simulink model "DC_Motor_Speed_Feedback_Controller"  (R2019b)
settings: Solver=FixedStepAuto  StartTime=0.0  StopTime=500  FixedStep=0.02  RelTol=1e-3  EnableMultiTasking=on
libraries: simulink x1, RoboholicLib x1, arduinolib x1
settings Model: SimulationMode=external  ExtModeTrigDuration=2  Creator=nbibin001  LastModifiedBy=ganna
settings DataIOCC: ReturnWorkspaceOutputs=off
settings OptimizationCC: PassReuseOutputArgsAs=Individual arguments  MaxStackSize=64  EfficientTunableParamExpr=on
settings DebuggingCC: ParameterTunabilityLossMsg=error  ArithmeticOperatorsInVariantConditions=warning
settings HardwareCC: ProdBitPerInt=16  ProdBitPerPointer=16  ProdBitPerSizeT=16  ProdBitPerPtrDiffT=16  ProdLargestAtomicFloat=None  ProdWordSize=8  ProdHWDeviceType=Atmel->AVR
settings SFSimCC: SimUseLocalCustomCode=off  MATLABDynamicMemAlloc=off  CustomCodeUndefinedFunction=UseInterfaceOnly
settings RTWCC: SystemTargetFile=ert.tlc  HardwareBoard=Arduino Mega 2560  TLCOptions=-aInlineSetEventsForThisBaseRateFcn=TLC_FALSE -aSuppressMultiTaskScheduler=TLC_FALSE -aRateBasedStepFcn=1  TemplateMakefile=ert_default_tmf  GenerateReport=on  RTWUseLocalCustomCode=off  Toolchain=Arduino AVR  BuildConfiguration=Faster Runs  IncludeHyperlinkInReport=on  LaunchReport=on  GenerateTraceInfo=on  GenerateTraceReport=on  GenerateTraceReportSl=on  GenerateTraceReportSf=on  GenerateTraceReportEml=on
settings CodeAppCC: ForceParamTrailComments=on  IgnoreCustomStorageClasses=off  OperatorAnnotations=on  SimulinkDataObjDesc=on  SFDataObjDesc=on  MATLABFcnDesc=on  InsertBlockDesc=on  StateflowObjectComments=on  MATLABSourceComments=on
settings ERTTargetCC: SupportContinuousTime=on  SupportNonInlinedSFcns=on  SupportVariableSizeSignals=on

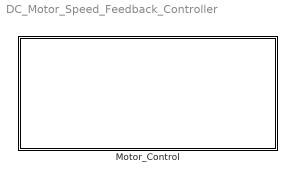
== system DC_Motor_Speed_Feedback_Controller ==
  Motor_Control : Subsystem  RTWFcnName=Motor_Control  RTWFileName=motor_control_file
      settings: RTWSystemCode=Nonreusable function  RTWFcnNameOpts=User specified  RTWFileNameOpts=User specified

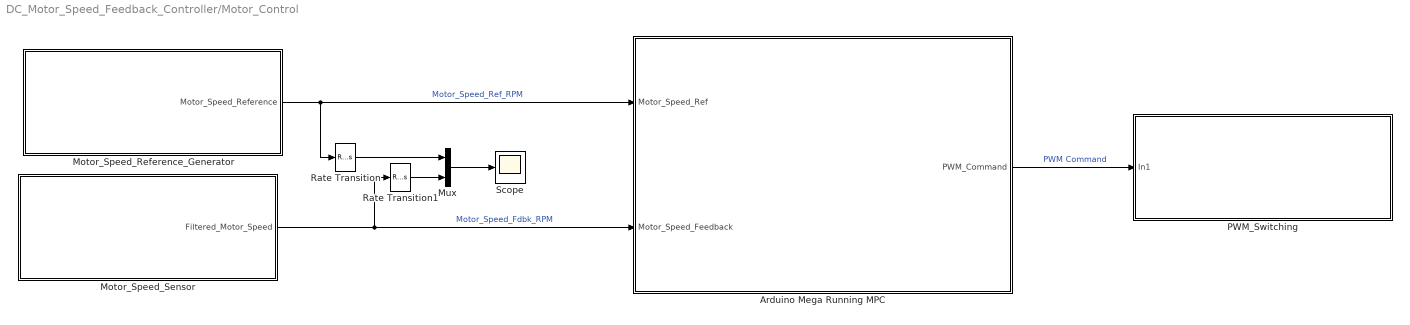
== system DC_Motor_Speed_Feedback_Controller/Motor_Control ==
  Arduino Mega Running MPC : Subsystem
      mask Display:
      | pic=imread('Chapter_9_Section_10_Controller_Image.jpg');
      | image(pic);
  Motor_Speed_Reference_Generator : Subsystem
      mask Display:
      | pic=imread('Chapter_9_Section_10_Speed_Ref_Figure.jpg');
      | image(pic);
  Motor_Speed_Sensor : Subsystem
      mask Display:
      | pic=imread('DC_Motor_with_Encoder.JPG');
      | image(pic);
  Mux : Mux  Inputs=2
  PWM_Switching : Subsystem
      mask Display:
      | pic=imread('Chapter_9_Section_10_PWM_Figure.jpg');
      | image(pic);
  Rate Transition : RateTransition
  Rate Transition1 : RateTransition
  Scope : Scope
  wires:
  Arduino Mega Running MPC/1(PWM_Command) -> PWM_Switching/1(In1)  "PWM Command"
  Motor_Speed_Sensor/1(Filtered_Motor_Speed) -> Rate Transition1/1, Arduino Mega Running MPC/2(Motor_Speed_Feedback)  "Motor_Speed_Fdbk_RPM"
  Motor_Speed_Reference_Generator/1(Motor_Speed_Reference) -> Rate Transition/1, Arduino Mega Running MPC/1(Motor_Speed_Ref)  "Motor_Speed_Ref_RPM"
  Rate Transition/1 -> Mux/1
  Rate Transition1/1 -> Mux/2
  Mux/1 -> Scope/1

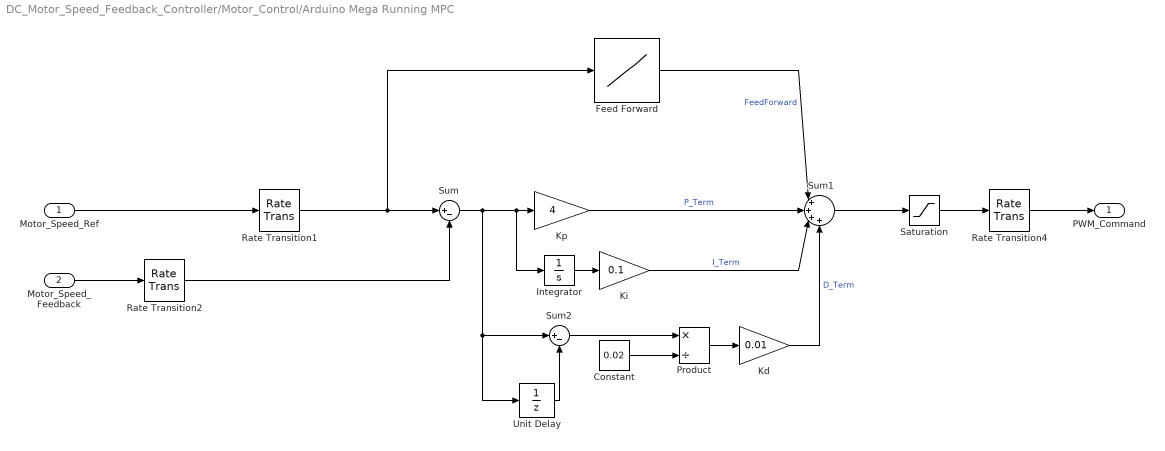
== system DC_Motor_Speed_Feedback_Controller/Motor_Control/Arduino Mega Running MPC ==
  Motor_Speed_Ref : Inport
  Motor_Speed_Feedback : Inport  Port=2
  Constant : Constant  Value=0.02
  Feed Forward : Lookup_n-D  NumberOfTableDimensions=1  BreakpointsForDimension1=[57 149 225 273 303 327 338 354 360 375]  Table="[25.5 \t50.1 \t76.5 \t102 \t127.5 \t153 \t178.5 \t204 \t229.5 \t255 ]"  ExtrapMethod=Clip  InternalRulePriority=Speed  RndMeth=Simplest  InputSameDT=on
  Integrator : Integrator
  Kd : Gain  Gain=0.01
  Ki : Gain  Gain=0.1
  "Kp " : Gain  Gain=4
  Product : Product  Inputs=*/
  Rate Transition1 : RateTransition
  Rate Transition2 : RateTransition
  Rate Transition4 : RateTransition
  Saturation : Saturate  UpperLimit=255  LowerLimit=0
  Sum : Sum  Inputs=|+-
  Sum1 : Sum  Inputs=|++++
  Sum2 : Sum  Inputs=|+-
  Unit Delay : UnitDelay  SampleTime=-1  HasFrameUpgradeWarning=on
  PWM_Command : Outport  VectorParamsAs1DForOutWhenUnconnected=off
  wires:
  Motor_Speed_Feedback/1 -> Rate Transition2/1
  Motor_Speed_Ref/1 -> Rate Transition1/1
  Rate Transition1/1 -> Feed Forward/1, Sum/1
  Rate Transition2/1 -> Sum/2
  Saturation/1 -> Rate Transition4/1
  Sum1/1 -> Saturation/1
  Integrator/1 -> Ki/1
  Sum/1 -> Unit Delay/1, Sum2/1, Integrator/1, "Kp "/1
  Feed Forward/1 -> Sum1/1  "FeedForward"
  "Kp "/1 -> Sum1/2  "P_Term"
  Ki/1 -> Sum1/3  "I_Term"
  Unit Delay/1 -> Sum2/2
  Sum2/1 -> Product/1
  Constant/1 -> Product/2
  Product/1 -> Kd/1
  Kd/1 -> Sum1/4  "D_Term"
  Rate Transition4/1 -> PWM_Command/1

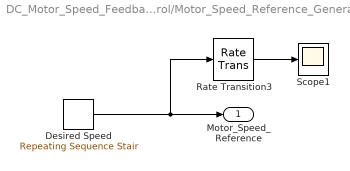
== system DC_Motor_Speed_Feedback_Controller/Motor_Control/Motor_Speed_Reference_Generator ==
  Desired Speed : simulink/Sources/Repeating Sequence Stair  OutValues=[110:200 199:-1:110]  tsamp=0.2  OutMin=[]  OutMax=[]  OutDataTypeStr=double  OutputDataTypeScalingMode=double  OutDataType=fixdt(0,8)  ConRadixGroup=Best Precision: Vector-wise  OutScaling=2^-12
  Rate Transition3 : RateTransition
  Scope1 : Scope
  Motor_Speed_Reference : Outport  VectorParamsAs1DForOutWhenUnconnected=off
  wires:
  Desired Speed/1 -> Rate Transition3/1, Motor_Speed_Reference/1
  Rate Transition3/1 -> Scope1/1

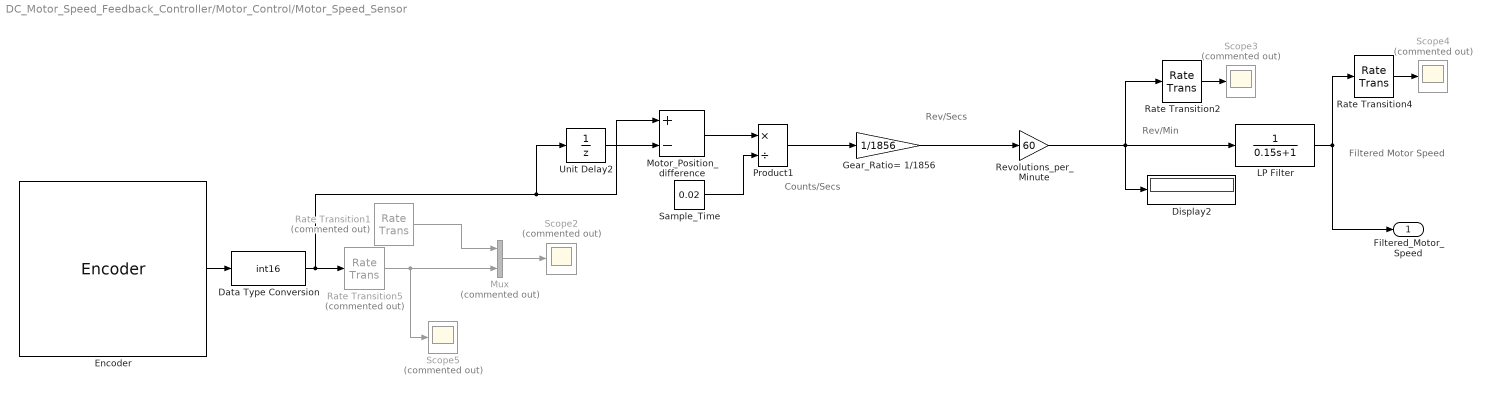
== system DC_Motor_Speed_Feedback_Controller/Motor_Control/Motor_Speed_Sensor ==
  note: Counts/Secs
  note: Rev/Secs
  note: Rev/Min
  note: Filtered Motor Speed
  Data Type Conversion : DataTypeConversion  OutDataTypeStr=int16
  Display2 : Display
  Encoder : RoboholicLib/Encoder  pinNumber1=5  pinNumber2=6
      settings: SourceProductName=Roboholic Maniacs Arduino Support Package
  Gear_Ratio= 1/1856 : Gain  Gain=1/1856
  LP Filter : TransferFcn  Denominator=[0.15 1]
  Motor_Position_difference : Sum  Inputs=+-
  Mux : Mux  Commented=on  Inputs=2
  Product1 : Product  Inputs=*/
  Rate Transition1 : RateTransition  Commented=on
  Rate Transition2 : RateTransition
  Rate Transition4 : RateTransition
  Rate Transition5 : RateTransition  Commented=on
  Revolutions_per_Minute : Gain  Gain=60
  Sample_Time : Constant  Value=0.02  OutDataTypeStr=double
  Scope{2..5} (4 alike) : Scope  Commented=on
  Unit Delay2 : UnitDelay  SampleTime=-1  HasFrameUpgradeWarning=on
  Filtered_Motor_Speed : Outport  VectorParamsAs1DForOutWhenUnconnected=off
  wires:
  Product1/1 -> Gear_Ratio= 1/1856/1
  Unit Delay2/1 -> Motor_Position_difference/2
  Rate Transition2/1 -> Scope3/1
  Rate Transition4/1 -> Scope4/1
  Motor_Position_difference/1 -> Product1/1
  Gear_Ratio= 1/1856/1 -> Revolutions_per_Minute/1
  Revolutions_per_Minute/1 -> LP Filter/1, Display2/1, Rate Transition2/1
  LP Filter/1 -> Rate Transition4/1, Filtered_Motor_Speed/1
  Sample_Time/1 -> Product1/2
  Encoder/1 -> Data Type Conversion/1
  Mux/1 -> Scope2/1
  Rate Transition1/1 -> Mux/1
  Rate Transition5/1 -> Scope5/1, Mux/2
  Data Type Conversion/1 -> Unit Delay2/1, Motor_Position_difference/1, Rate Transition5/1

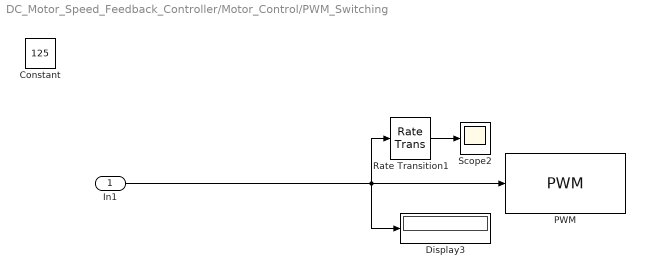
== system DC_Motor_Speed_Feedback_Controller/Motor_Control/PWM_Switching ==
  In1 : Inport
  Constant : Constant  Value=125
  Display3 : Display
  PWM : arduinolib/PWM  pinNumber=5  EnableInputFrequency=off  InitialFrequency=2000  InitialDutyCycle=0  NotificationType=None  blockPlatform=arduino
  Rate Transition1 : RateTransition
  Scope2 : Scope
  wires:
  Rate Transition1/1 -> Scope2/1
  In1/1 -> PWM/1, Rate Transition1/1, Display3/1
